simulink model "iwave_dsa_1ant"  (R2019a)
settings: Solver=VariableStepAuto  StartTime=0.0  StopTime=10.0  RelTol=1e-3
undefined symbols (not defined in the file): i
libraries: xbsIndex_r4 x9262, casper_library_misc x249, xps_library x3, casper_library_reorder x2, casper_library_delays x2
(part 15 of 96)

== system iwave_dsa_1ant/pipeline0/input/bus_mux ==
  sel : Inport
  d0 : Inport  Port=2
  d1 : Inport  Port=3
  d2 : Inport  Port=4
  misci : Inport  Port=5
  d_bussify : Subsystem  AncestorBlock=casper_library_flow_control/bus_create  mask(bus_create){inputNum=4}
      mask prompts: inputNum "Number of inputs:"
      mask init:
      | bus_create_init(gcb,...
      |     'inputNum', inputNum);
  dmisc : xbsIndex_r4/Delay  rst=off  infoeditControl=Selection of Reset will increase slice count due to use of real FFs and instead of SRLs  en=off  latency=1  reg_retiming=on  dbl_ovrd=off  block_type=delay
  expand0 : Subsystem  AncestorBlock=casper_library_flow_control/bus_expand  mask(bus_expand){mode=divisions of arbitrary size, outputNum=1, outputWidth=[192;192;192;192], outputBinaryPt=[0  0  0  0], outputArithmeticType=[0  0  0  0], show_format=on, outputToWorkspace=off, variablePrefix=, outputToModelAsWell=on}
      mask prompts: outputNum "Number of outputs:"; outputWidth "Output width [msb ... lsb]:"; outputBinaryPt "Output binary point position [msb ... lsb]:"; outputArithmeticType "Output arithmetic type (ufix=0, fix=1, bool=2) [msb ... lsb]:"; show_format "Print format string?"; outputToWorkspace "Output to workspace?"; variablePrefix "Variable name prefix:"; outputToModelAsWell "Output to model as well?"
      mask help:
      | Expands a 'bus' made using a bus_create or Xilinx
      | concat block.
      | The input will be divided into the specified number
      | of outputs with the specified arithmetic types.
      | Divisions are made from most significant bit.
      mask init: same as iwave_dsa_1ant/pipeline0/bus_expand
      settings: AttributesFormatString=4 outputs: uf192.0,uf192.0,uf192.0,uf192.0,
      mask TypeOptions mode: divisions of equal size | divisions of arbitrary size
      mask Callback mode: bus_expand_callback();
      mask Callback outputWidth: bus_expand_callback();
      mask Callback outputToWorkspace: bus_expand_callback();
  expand1 : Subsystem  AncestorBlock=casper_library_flow_control/bus_expand  mask(bus_expand){mode=divisions of arbitrary size, outputNum=1, outputWidth=[192;192;192;192], outputBinaryPt=[0  0  0  0], outputArithmeticType=[0  0  0  0], show_format=on, outputToWorkspace=off, variablePrefix=, outputToModelAsWell=on}
      mask prompts: outputNum "Number of outputs:"; outputWidth "Output width [msb ... lsb]:"; outputBinaryPt "Output binary point position [msb ... lsb]:"; outputArithmeticType "Output arithmetic type (ufix=0, fix=1, bool=2) [msb ... lsb]:"; show_format "Print format string?"; outputToWorkspace "Output to workspace?"; variablePrefix "Variable name prefix:"; outputToModelAsWell "Output to model as well?"
      mask help:
      | Expands a 'bus' made using a bus_create or Xilinx
      | concat block.
      | The input will be divided into the specified number
      | of outputs with the specified arithmetic types.
      | Divisions are made from most significant bit.
      mask init: same as iwave_dsa_1ant/pipeline0/bus_expand
      settings: AttributesFormatString=4 outputs: uf192.0,uf192.0,uf192.0,uf192.0,
      mask TypeOptions mode: divisions of equal size | divisions of arbitrary size
      mask Callback mode: bus_expand_callback();
      mask Callback outputWidth: bus_expand_callback();
      mask Callback outputToWorkspace: bus_expand_callback();
  expand2 : Subsystem  AncestorBlock=casper_library_flow_control/bus_expand  mask(bus_expand){mode=divisions of arbitrary size, outputNum=1, outputWidth=[192;192;192;192], outputBinaryPt=[0  0  0  0], outputArithmeticType=[0  0  0  0], show_format=on, outputToWorkspace=off, variablePrefix=, outputToModelAsWell=on}
      mask prompts: outputNum "Number of outputs:"; outputWidth "Output width [msb ... lsb]:"; outputBinaryPt "Output binary point position [msb ... lsb]:"; outputArithmeticType "Output arithmetic type (ufix=0, fix=1, bool=2) [msb ... lsb]:"; show_format "Print format string?"; outputToWorkspace "Output to workspace?"; variablePrefix "Variable name prefix:"; outputToModelAsWell "Output to model as well?"
      mask help:
      | Expands a 'bus' made using a bus_create or Xilinx
      | concat block.
      | The input will be divided into the specified number
      | of outputs with the specified arithmetic types.
      | Divisions are made from most significant bit.
      mask init: same as iwave_dsa_1ant/pipeline0/bus_expand
      settings: AttributesFormatString=4 outputs: uf192.0,uf192.0,uf192.0,uf192.0,
      mask TypeOptions mode: divisions of equal size | divisions of arbitrary size
      mask Callback mode: bus_expand_callback();
      mask Callback outputWidth: bus_expand_callback();
      mask Callback outputToWorkspace: bus_expand_callback();
  mux{0..3} (4 alike) : xbsIndex_r4/Mux  inputs=3  en=off  latency=1  precision=Full  arith_type=Unsigned  n_bits=16  bin_pt=14  quantization=Truncate  overflow=Wrap  dbl_ovrd=off  block_type=mux
  sel_expand : Subsystem  AncestorBlock=casper_library_flow_control/bus_expand  mask(bus_expand){mode=divisions of equal size, outputNum=4, outputWidth=2, outputBinaryPt=0, outputArithmeticType=0, show_format=on, outputToWorkspace=off, variablePrefix=, outputToModelAsWell=on}
      mask prompts: outputNum "Number of outputs:"; outputWidth "Output width:"; outputBinaryPt "Output binary point position:"; outputArithmeticType "Output arithmetic type (ufix=0, fix=1, bool=2):"; show_format "Print format string?"; outputToWorkspace "Output to workspace?"; variablePrefix "Variable name prefix:"; outputToModelAsWell "Output to model as well?"
      mask help:
      | Expands a 'bus' made using a bus_create or Xilinx
      | concat block.
      | The input will be divided into the specified number
      | of outputs with the specified arithmetic types.
      | Divisions are made from most significant bit.
      mask init: same as iwave_dsa_1ant/pipeline0/bus_expand
      settings: AttributesFormatString=4 outputs: uf2.0,uf2.0,uf2.0,uf2.0,
      mask TypeOptions mode: divisions of equal size | divisions of arbitrary size
      mask Callback mode: bus_expand_callback();
      mask Callback outputWidth: bus_expand_callback();
      mask Callback outputToWorkspace: bus_expand_callback();
  out : Outport
  misco : Outport  Port=2
  wires:
  sel/1 -> sel_expand/1(bus_in)
  d0/1 -> expand0/1(bus_in)
  d1/1 -> expand1/1(bus_in)
  d2/1 -> expand2/1(bus_in)
  sel_expand/1(msb_out4) -> mux0/1
  expand0/1(msb_out4) -> mux0/2
  expand1/1(msb_out4) -> mux0/3
  expand2/1(msb_out4) -> mux0/4
  sel_expand/2(out3) -> mux1/1
  expand0/2(out3) -> mux1/2
  expand1/2(out3) -> mux1/3
  expand2/2(out3) -> mux1/4
  sel_expand/3(out2) -> mux2/1
  expand0/3(out2) -> mux2/2
  expand1/3(out2) -> mux2/3
  expand2/3(out2) -> mux2/4
  sel_expand/4(lsb_out1) -> mux3/1
  expand0/4(lsb_out1) -> mux3/2
  expand1/4(lsb_out1) -> mux3/3
  expand2/4(lsb_out1) -> mux3/4
  misci/1 -> dmisc/1
  mux0/1 -> d_bussify/1(in1)
  mux1/1 -> d_bussify/2(in2)
  mux2/1 -> d_bussify/3(in3)
  mux3/1 -> d_bussify/4(in4)
  d_bussify/1(bus_out) -> out/1
  dmisc/1 -> misco/1

== system iwave_dsa_1ant/pipeline0/input/rms ==
  note: two clocks after
      | adc_rms_rst goes high
      | the outputs are locked
  note: To provide a means for measuring the magnitude of the signals
      | coming in to each ADC channel, we have a "calc_adc_sum_sq"
      | block which uses a single multiplier, two accumulators, and two
      | regsiters to calculate the sum of 64K ADC samples and the sum
      | of squares of 64K ADC samples.  These can be used to calculate
      | the mean (aka DC offset) and standard deviation (aka RMS) of
      | the ADC inputs.
  note: The sum_sumsq values are Fix_64_0.
      | The upper 29 bits are Fix_29_0 sum of samples.
      | The lower 35 bits are UFix_35_0 sum of squares.
  note: sum,sq,sum,sq,...
  in : Inport
  Constant : Constant  Value=0
  Counter : xbsIndex_r4/Counter  cnt_type=Free Running  cnt_to=Inf  operation=Up  start_count=0  cnt_by_val=1  arith_type=Unsigned  n_bits=16  bin_pt=0  load_pin=off  rst=off  en=off  explicit_period=off  period=1  use_behavioral_HDL=off  implementation=Fabric  use_rpm=on  dbl_ovrd=off  block_type=counter
      settings: xl_area=[0, 0, 0, 0, 0, 0, 0]
  Goto Tag Visibility : GotoTagVisibility  GotoTag=adc_rms_rst
  Slice16 : xbsIndex_r4/Slice  nbits=1  boolean_output=on  mode=Upper Bit Location + Width  bit1=0  base1=MSB of Input  bit0=19  base0=LSB of Input  dbl_ovrd=off  block_type=slice
      settings: infoedit="Extracts a given range of bits from each input sample and presents it at the output.  The output type is ordinarily unsigned with binary point at zero, but can be Boolean when the slice is one bit wide.<P><P>Hardware notes: In hardware this block costs nothing."  block_version=10.1.3
  Subsystem : Subsystem
  Subsystem1 : Subsystem
  Subsystem2 : Subsystem
  Subsystem3 : Subsystem
  Terminator : Terminator
  bram_ctrl : Subsystem
  bus_expand : Subsystem  AncestorBlock=casper_library_flow_control/bus_expand  mask(bus_expand){mode=divisions of equal size, outputNum=8*16, outputWidth=3, outputBinaryPt=0, outputArithmeticType=1, show_format=off, outputToWorkspace=off, variablePrefix=out, outputToModelAsWell=on}
      mask prompts: outputNum "Number of outputs:"; outputWidth "Output width:"; outputBinaryPt "Output binary point position:"; outputArithmeticType "Output arithmetic type (ufix=0, fix=1, bool=2):"; show_format "Print format string?"; outputToWorkspace "Output to workspace?"; variablePrefix "Variable name prefix:"; outputToModelAsWell "Output to model as well?"
      mask help:
      | Expands a 'bus' made using a bus_create or Xilinx
      | concat block.
      | The input will be divided into the specified number
      | of outputs with the specified arithmetic types.
      | Divisions are made from most significant bit.
      mask init: same as iwave_dsa_1ant/pipeline0/bus_expand
      settings: AttributesFormatString=128 outputs
      mask TypeOptions mode: divisions of equal size | divisions of arbitrary size
      mask Callback mode: bus_expand_callback();
      mask Callback outputWidth: bus_expand_callback();
      mask Callback outputToWorkspace: bus_expand_callback();
  edge_detect : Subsystem  AncestorBlock=casper_library_misc/edge_detect  mask(edge_detect){edge=Rising, polarity=Active High, x_in=[0 0.08 0.08 0.16 0.16 0.24 0.24 0.32 0.32 0.4], y_in=[-1 -1  1  1  1  1  1  1  1  1], x_out=[0.6 0.68 0.68 0.76 0.76 0.84 0.84 0.92 0.92 1], y_out=[-1 -1  1  1 -1 -1 -1 -1 -1 -1]}
      mask prompts: edge "Edge Type"; polarity "Output Polarity"; x_in "Input X Positions"; y_in "Input Y Positions"; x_out "Output X Positions"; y_out "Output Y Positions"
      mask help: Output is active for one-cycle after each edge of the specified type (i.e. rising, falling or both).
      mask init: same as iwave_dsa_1ant/pipeline0/sync/ed1
      settings: AttributesFormatString=|
      | rising edges
      | active high
      mask Help: Output is active for one-cycle after each edge of the specified type (i.e. rising, falling, or both).  Latency is zero.
      mask TypeOptions edge: Rising | Falling | Both
      mask TypeOptions polarity: Active High | Active Low
      mask Display:
      | plot(x_in_num,0.5+y_in_num*0.2);
      | plot(x_out_num,0.5+y_out_num*0.2);
  enable : Subsystem  Tag=xps:sw_reg  AncestorBlock=xps_library/Memory/software_register  mask(swreg){io_dir=From Processor, io_delay=0, init_val=0, sample_period=1, names=reg, bitwidths=32, bin_pts=0, arith_types=0, sim_port=on, show_format=off, desc_str=|}
      mask desc_str=|
      | Enable statistics recording. If the least-significant bit
      | is ``1``, statistics will be recorded to RAM.
      mask prompts: io_dir "I/O direction"; io_delay "I/O delay"; init_val "Initial Value"; sample_period "Sample period"; names "Bitfield names [msb...lsb]"; bitwidths "Bitfield widths"; bin_pts "Bitfield binary pts"; arith_types "Bitfield types, ufix=0, fix=1, bool=2"; sim_port "Provide sim input/output?"; show_format "Print format string?"; desc_str "Description"
      mask help: A 32-bit software-accessible register. Can be divided into bitfields of varying widths and types using the fields in the block mask.
      mask init:
      | swreg_init(gcb)
      settings: AttributesFormatString=1input
      mask TypeOptions io_dir: To Processor | From Processor
      mask Callback io_dir:
      | mask_enables = get_param(gcb, 'MaskEnables');
      | mask_names = get_param(gcb, 'MaskNames');
      | if strcmp(get_param(gcb, 'io_dir'), 'To Processor'),
      |     mask_enables{ismember(mask_names, 'sample_period')} = 'off';
      | else
      |     mask_enables{ismember(mask_names, 'sample_period')} = 'on';
      | end
      | set_param(gcb, 'MaskEnables', mask_enables);
      mask DialogControl ParameterTabVar0 Prompt: Setup
  levels : Subsystem  Tag=xps:bram  AncestorBlock=xps_library/Memory/shared_bram  mask{sample_rate=1, init_vals=[0:2^10-1], data_bin_pt=0, optimization=Minimum_Area, reg_core_output=on, reg_prim_output=on, data_width=64, addr_width=9, arith_type=Unsigned, desc_str=|, type_desc=uint64}
      mask desc_str=|
      | Multi-channel statistics. For the ``n`` th 64-bit word, the
      | least signficant 32 bits represent the accumulated
      | ADC power, accumulated over 65536 samples and
      | stored as an unsigned 32-bit integer.
      | The most significant 32 bits represent the sum of
      | 65536 ADC samples stored as a signed 32-bit integer.
      mask prompts: sample_rate "Sample rate"; init_vals "Initial values (simulation only)"; data_bin_pt "Data Binary Point"; reg_core_output "Register Core Output"; reg_prim_output "Register Primitive Output"; data_width "Data Width"; addr_width "Address width"; arith_type "Output Data Type"; desc_str "Description"; type_desc "Word Type Description"
      mask init:
      | shared_bram_mask;
      mask TypeOptions optimization: Minimum_Area | Low_Power
      mask TypeOptions data_width: 8 | 16 | 32 | 64 | 128
      mask TypeOptions arith_type: Unsigned | Signed  (2's comp)
      mask DialogControl Container4 Prompt: Configuration
      mask DialogControl Container10 Prompt: Documentation
  lsb : xbsIndex_r4/Slice  nbits=0  boolean_output=on  mode=Lower Bit Location + Width  bit1=0  base1=MSB of Input  bit0=0  base0=LSB of Input  dbl_ovrd=off  block_type=slice
      settings: block_version=10.1.3
  tag scope: adc_rms_rst=scoped
  wires:
  Counter/1 -> Slice16/1
  Slice16/1 -> edge_detect/1(in)
  edge_detect/1(out) -> [adc_rms_rst]
  enable/1(in_reg) -> lsb/1
  bram_ctrl/1(addr) -> levels/1(addr)
  bram_ctrl/2(data) -> levels/2(data_in)
  bram_ctrl/3(we) -> levels/3(we)
  Constant/1 -> enable/1(sim_1)
  levels/1(data_out) -> Terminator/1
  in/1 -> bus_expand/1(bus_in)
  lsb/1 -> bram_ctrl/1(en)
  Subsystem/1(Out1) -> bram_ctrl/2(adc0)
  Subsystem/2(Out2) -> bram_ctrl/3(adc1)
  Subsystem/3(Out3) -> bram_ctrl/4(adc2)
  Subsystem/4(Out4) -> bram_ctrl/5(adc3)
  Subsystem/5(Out5) -> bram_ctrl/6(adc4)
  Subsystem/6(Out6) -> bram_ctrl/7(adc5)
  Subsystem/7(Out7) -> bram_ctrl/8(adc6)
  Subsystem/8(Out8) -> bram_ctrl/9(adc7)
  Subsystem/9(Out9) -> bram_ctrl/10(adc8)
  Subsystem/10(Out10) -> bram_ctrl/11(adc9)
  Subsystem/11(Out11) -> bram_ctrl/12(adc10)
  Subsystem/12(Out12) -> bram_ctrl/13(adc11)
  Subsystem/13(Out13) -> bram_ctrl/14(adc12)
  Subsystem/14(Out14) -> bram_ctrl/15(adc13)
  Subsystem/15(Out15) -> bram_ctrl/16(adc14)
  Subsystem/16(Out16) -> bram_ctrl/17(adc15)
  Subsystem/17(Out17) -> bram_ctrl/18(adc16)
  Subsystem/18(Out18) -> bram_ctrl/19(adc17)
  Subsystem/19(Out19) -> bram_ctrl/20(adc18)
  Subsystem/20(Out20) -> bram_ctrl/21(adc19)
  Subsystem/21(Out21) -> bram_ctrl/22(adc20)
  Subsystem/22(Out22) -> bram_ctrl/23(adc21)
  Subsystem/23(Out23) -> bram_ctrl/24(adc22)
  Subsystem/24(Out24) -> bram_ctrl/25(adc23)
  Subsystem/25(Out25) -> bram_ctrl/26(adc24)
  Subsystem/26(Out26) -> bram_ctrl/27(adc25)
  Subsystem/27(Out27) -> bram_ctrl/28(adc26)
  Subsystem/28(Out28) -> bram_ctrl/29(adc27)
  Subsystem/29(Out29) -> bram_ctrl/30(adc28)
  Subsystem/30(Out30) -> bram_ctrl/31(adc29)
  Subsystem/31(Out31) -> bram_ctrl/32(adc30)
  Subsystem/32(Out32) -> bram_ctrl/33(adc31)
  bus_expand/1(msb_out128) -> Subsystem/1(In1)
  bus_expand/2(out127) -> Subsystem/2(In2)
  bus_expand/3(out126) -> Subsystem/3(In3)
  bus_expand/4(out125) -> Subsystem/4(In4)
  bus_expand/5(out124) -> Subsystem/5(In5)
  bus_expand/6(out123) -> Subsystem/6(In6)
  bus_expand/7(out122) -> Subsystem/7(In7)
  bus_expand/8(out121) -> Subsystem/8(In8)
  bus_expand/9(out120) -> Subsystem/9(In9)
  bus_expand/10(out119) -> Subsystem/10(In10)
  bus_expand/11(out118) -> Subsystem/11(In11)
  bus_expand/12(out117) -> Subsystem/12(In12)
  bus_expand/13(out116) -> Subsystem/13(In13)
  bus_expand/14(out115) -> Subsystem/14(In14)
  bus_expand/15(out114) -> Subsystem/15(In15)
  bus_expand/16(out113) -> Subsystem/16(In16)
  bus_expand/17(out112) -> Subsystem/17(In17)
  bus_expand/18(out111) -> Subsystem/18(In18)
  bus_expand/19(out110) -> Subsystem/19(In19)
  bus_expand/20(out109) -> Subsystem/20(In20)
  bus_expand/21(out108) -> Subsystem/21(In21)
  bus_expand/22(out107) -> Subsystem/22(In22)
  bus_expand/23(out106) -> Subsystem/23(In23)
  bus_expand/24(out105) -> Subsystem/24(In24)
  bus_expand/25(out104) -> Subsystem/25(In25)
  bus_expand/26(out103) -> Subsystem/26(In26)
  bus_expand/27(out102) -> Subsystem/27(In27)
  bus_expand/28(out101) -> Subsystem/28(In28)
  bus_expand/29(out100) -> Subsystem/29(In29)
  bus_expand/30(out99) -> Subsystem/30(In30)
  bus_expand/31(out98) -> Subsystem/31(In31)
  bus_expand/32(out97) -> Subsystem/32(In32)
  bus_expand/33(out96) -> Subsystem1/1(In1)
  bus_expand/34(out95) -> Subsystem1/2(In2)
  bus_expand/35(out94) -> Subsystem1/3(In3)
  bus_expand/36(out93) -> Subsystem1/4(In4)
  bus_expand/37(out92) -> Subsystem1/5(In5)
  bus_expand/38(out91) -> Subsystem1/6(In6)
  bus_expand/39(out90) -> Subsystem1/7(In7)
  bus_expand/40(out89) -> Subsystem1/8(In8)
  bus_expand/41(out88) -> Subsystem1/9(In9)
  bus_expand/42(out87) -> Subsystem1/10(In10)
  bus_expand/43(out86) -> Subsystem1/11(In11)
  bus_expand/44(out85) -> Subsystem1/12(In12)
  bus_expand/45(out84) -> Subsystem1/13(In13)
  bus_expand/46(out83) -> Subsystem1/14(In14)
  bus_expand/47(out82) -> Subsystem1/15(In15)
  bus_expand/48(out81) -> Subsystem1/16(In16)
  bus_expand/49(out80) -> Subsystem1/17(In17)
  bus_expand/50(out79) -> Subsystem1/18(In18)
  bus_expand/51(out78) -> Subsystem1/19(In19)
  bus_expand/52(out77) -> Subsystem1/20(In20)
  bus_expand/53(out76) -> Subsystem1/21(In21)
  bus_expand/54(out75) -> Subsystem1/22(In22)
  bus_expand/55(out74) -> Subsystem1/23(In23)
  bus_expand/56(out73) -> Subsystem1/24(In24)
  bus_expand/57(out72) -> Subsystem1/25(In25)
  bus_expand/58(out71) -> Subsystem1/26(In26)
  bus_expand/59(out70) -> Subsystem1/27(In27)
  bus_expand/60(out69) -> Subsystem1/28(In28)
  bus_expand/61(out68) -> Subsystem1/29(In29)
  bus_expand/62(out67) -> Subsystem1/30(In30)
  bus_expand/63(out66) -> Subsystem1/31(In31)
  bus_expand/64(out65) -> Subsystem1/32(In32)
  Subsystem1/1(Out1) -> bram_ctrl/34(adc32)
  Subsystem1/2(Out2) -> bram_ctrl/35(adc33)
  Subsystem1/3(Out3) -> bram_ctrl/36(adc34)
  Subsystem1/4(Out4) -> bram_ctrl/37(adc35)
  Subsystem1/5(Out5) -> bram_ctrl/38(adc36)
  Subsystem1/6(Out6) -> bram_ctrl/39(adc37)
  Subsystem1/7(Out7) -> bram_ctrl/40(adc38)
  Subsystem1/8(Out8) -> bram_ctrl/41(adc39)
  Subsystem1/9(Out9) -> bram_ctrl/42(adc40)
  Subsystem1/10(Out10) -> bram_ctrl/43(adc41)
  Subsystem1/11(Out11) -> bram_ctrl/44(adc42)
  Subsystem1/12(Out12) -> bram_ctrl/45(adc43)
  Subsystem1/13(Out13) -> bram_ctrl/46(adc44)
  Subsystem1/14(Out14) -> bram_ctrl/47(adc45)
  Subsystem1/15(Out15) -> bram_ctrl/48(adc46)
  Subsystem1/16(Out16) -> bram_ctrl/49(adc47)
  Subsystem1/17(Out17) -> bram_ctrl/50(adc48)
  Subsystem1/18(Out18) -> bram_ctrl/51(adc49)
  Subsystem1/19(Out19) -> bram_ctrl/52(adc50)
  Subsystem1/20(Out20) -> bram_ctrl/53(adc51)
  Subsystem1/21(Out21) -> bram_ctrl/54(adc52)
  Subsystem1/22(Out22) -> bram_ctrl/55(adc53)
  Subsystem1/23(Out23) -> bram_ctrl/56(adc54)
  Subsystem1/24(Out24) -> bram_ctrl/57(adc55)
  Subsystem1/25(Out25) -> bram_ctrl/58(adc56)
  Subsystem1/26(Out26) -> bram_ctrl/59(adc57)
  Subsystem1/27(Out27) -> bram_ctrl/60(adc58)
  Subsystem1/28(Out28) -> bram_ctrl/61(adc59)
  Subsystem1/29(Out29) -> bram_ctrl/62(adc60)
  Subsystem1/30(Out30) -> bram_ctrl/63(adc61)
  Subsystem1/31(Out31) -> bram_ctrl/64(adc62)
  Subsystem1/32(Out32) -> bram_ctrl/65(adc63)
  bus_expand/65(out64) -> Subsystem2/1(In1)
  bus_expand/66(out63) -> Subsystem2/2(In2)
  bus_expand/67(out62) -> Subsystem2/3(In3)
  bus_expand/68(out61) -> Subsystem2/4(In4)
  bus_expand/69(out60) -> Subsystem2/5(In5)
  bus_expand/70(out59) -> Subsystem2/6(In6)
  bus_expand/71(out58) -> Subsystem2/7(In7)
  bus_expand/72(out57) -> Subsystem2/8(In8)
  bus_expand/73(out56) -> Subsystem2/9(In9)
  bus_expand/74(out55) -> Subsystem2/10(In10)
  bus_expand/75(out54) -> Subsystem2/11(In11)
  bus_expand/76(out53) -> Subsystem2/12(In12)
  bus_expand/77(out52) -> Subsystem2/13(In13)
  bus_expand/78(out51) -> Subsystem2/14(In14)
  bus_expand/79(out50) -> Subsystem2/15(In15)
  bus_expand/80(out49) -> Subsystem2/16(In16)
  bus_expand/81(out48) -> Subsystem2/17(In17)
  bus_expand/82(out47) -> Subsystem2/18(In18)
  bus_expand/83(out46) -> Subsystem2/19(In19)
  bus_expand/84(out45) -> Subsystem2/20(In20)
  bus_expand/85(out44) -> Subsystem2/21(In21)
  bus_expand/86(out43) -> Subsystem2/22(In22)
  bus_expand/87(out42) -> Subsystem2/23(In23)
  bus_expand/88(out41) -> Subsystem2/24(In24)
  bus_expand/89(out40) -> Subsystem2/25(In25)
  bus_expand/90(out39) -> Subsystem2/26(In26)
  bus_expand/91(out38) -> Subsystem2/27(In27)
  bus_expand/92(out37) -> Subsystem2/28(In28)
  bus_expand/93(out36) -> Subsystem2/29(In29)
  bus_expand/94(out35) -> Subsystem2/30(In30)
  bus_expand/95(out34) -> Subsystem2/31(In31)
  bus_expand/96(out33) -> Subsystem2/32(In32)
  Subsystem2/1(Out1) -> bram_ctrl/66(adc64)
  Subsystem2/2(Out2) -> bram_ctrl/67(adc65)
  Subsystem2/3(Out3) -> bram_ctrl/68(adc66)
  Subsystem2/4(Out4) -> bram_ctrl/69(adc67)
  Subsystem2/5(Out5) -> bram_ctrl/70(adc68)
  Subsystem2/6(Out6) -> bram_ctrl/71(adc69)
  Subsystem2/7(Out7) -> bram_ctrl/72(adc70)
  Subsystem2/8(Out8) -> bram_ctrl/73(adc71)
  Subsystem2/9(Out9) -> bram_ctrl/74(adc72)
  Subsystem2/10(Out10) -> bram_ctrl/75(adc73)
  Subsystem2/11(Out11) -> bram_ctrl/76(adc74)
  Subsystem2/12(Out12) -> bram_ctrl/77(adc75)
  Subsystem2/13(Out13) -> bram_ctrl/78(adc76)
  Subsystem2/14(Out14) -> bram_ctrl/79(adc77)
  Subsystem2/15(Out15) -> bram_ctrl/80(adc78)
  Subsystem2/16(Out16) -> bram_ctrl/81(adc79)
  Subsystem2/17(Out17) -> bram_ctrl/82(adc80)
  Subsystem2/18(Out18) -> bram_ctrl/83(adc81)
  Subsystem2/19(Out19) -> bram_ctrl/84(adc82)
  Subsystem2/20(Out20) -> bram_ctrl/85(adc83)
  Subsystem2/21(Out21) -> bram_ctrl/86(adc84)
  Subsystem2/22(Out22) -> bram_ctrl/87(adc85)
  Subsystem2/23(Out23) -> bram_ctrl/88(adc86)
  Subsystem2/24(Out24) -> bram_ctrl/89(adc87)
  Subsystem2/25(Out25) -> bram_ctrl/90(adc88)
  Subsystem2/26(Out26) -> bram_ctrl/91(adc89)
  Subsystem2/27(Out27) -> bram_ctrl/92(adc90)
  Subsystem2/28(Out28) -> bram_ctrl/93(adc91)
  Subsystem2/29(Out29) -> bram_ctrl/94(adc92)
  Subsystem2/30(Out30) -> bram_ctrl/95(adc93)
  Subsystem2/31(Out31) -> bram_ctrl/96(adc94)
  Subsystem2/32(Out32) -> bram_ctrl/97(adc95)
  bus_expand/97(out32) -> Subsystem3/1(In1)
  bus_expand/98(out31) -> Subsystem3/2(In2)
  bus_expand/99(out30) -> Subsystem3/3(In3)
  bus_expand/100(out29) -> Subsystem3/4(In4)
  bus_expand/101(out28) -> Subsystem3/5(In5)
  bus_expand/102(out27) -> Subsystem3/6(In6)
  bus_expand/103(out26) -> Subsystem3/7(In7)
  bus_expand/104(out25) -> Subsystem3/8(In8)
  bus_expand/105(out24) -> Subsystem3/9(In9)
  bus_expand/106(out23) -> Subsystem3/10(In10)
  bus_expand/107(out22) -> Subsystem3/11(In11)
  bus_expand/108(out21) -> Subsystem3/12(In12)
  bus_expand/109(out20) -> Subsystem3/13(In13)
  bus_expand/110(out19) -> Subsystem3/14(In14)
  bus_expand/111(out18) -> Subsystem3/15(In15)
  bus_expand/112(out17) -> Subsystem3/16(In16)
  bus_expand/113(out16) -> Subsystem3/17(In17)
  bus_expand/114(out15) -> Subsystem3/18(In18)
  bus_expand/115(out14) -> Subsystem3/19(In19)
  bus_expand/116(out13) -> Subsystem3/20(In20)
  bus_expand/117(out12) -> Subsystem3/21(In21)
  bus_expand/118(out11) -> Subsystem3/22(In22)
  bus_expand/119(out10) -> Subsystem3/23(In23)
  bus_expand/120(out9) -> Subsystem3/24(In24)
  bus_expand/121(out8) -> Subsystem3/25(In25)
  bus_expand/122(out7) -> Subsystem3/26(In26)
  bus_expand/123(out6) -> Subsystem3/27(In27)
  bus_expand/124(out5) -> Subsystem3/28(In28)
  bus_expand/125(out4) -> Subsystem3/29(In29)
  bus_expand/126(out3) -> Subsystem3/30(In30)
  bus_expand/127(out2) -> Subsystem3/31(In31)
  bus_expand/128(lsb_out1) -> Subsystem3/32(In32)
  Subsystem3/1(Out1) -> bram_ctrl/98(adc96)
  Subsystem3/2(Out2) -> bram_ctrl/99(adc97)
  Subsystem3/3(Out3) -> bram_ctrl/100(adc98)
  Subsystem3/4(Out4) -> bram_ctrl/101(adc99)
  Subsystem3/5(Out5) -> bram_ctrl/102(adc100)
  Subsystem3/6(Out6) -> bram_ctrl/103(adc101)
  Subsystem3/7(Out7) -> bram_ctrl/104(adc102)
  Subsystem3/8(Out8) -> bram_ctrl/105(adc103)
  Subsystem3/9(Out9) -> bram_ctrl/106(adc104)
  Subsystem3/10(Out10) -> bram_ctrl/107(adc105)
  Subsystem3/11(Out11) -> bram_ctrl/108(adc106)
  Subsystem3/12(Out12) -> bram_ctrl/109(adc107)
  Subsystem3/13(Out13) -> bram_ctrl/110(adc108)
  Subsystem3/14(Out14) -> bram_ctrl/111(adc109)
  Subsystem3/15(Out15) -> bram_ctrl/112(adc110)
  Subsystem3/16(Out16) -> bram_ctrl/113(adc111)
  Subsystem3/17(Out17) -> bram_ctrl/114(adc112)
  Subsystem3/18(Out18) -> bram_ctrl/115(adc113)
  Subsystem3/19(Out19) -> bram_ctrl/116(adc114)
  Subsystem3/20(Out20) -> bram_ctrl/117(adc115)
  Subsystem3/21(Out21) -> bram_ctrl/118(adc116)
  Subsystem3/22(Out22) -> bram_ctrl/119(adc117)
  Subsystem3/23(Out23) -> bram_ctrl/120(adc118)
  Subsystem3/24(Out24) -> bram_ctrl/121(adc119)
  Subsystem3/25(Out25) -> bram_ctrl/122(adc120)
  Subsystem3/26(Out26) -> bram_ctrl/123(adc121)
  Subsystem3/27(Out27) -> bram_ctrl/124(adc122)
  Subsystem3/28(Out28) -> bram_ctrl/125(adc123)
  Subsystem3/29(Out29) -> bram_ctrl/126(adc124)
  Subsystem3/30(Out30) -> bram_ctrl/127(adc125)
  Subsystem3/31(Out31) -> bram_ctrl/128(adc126)
  Subsystem3/32(Out32) -> bram_ctrl/129(adc127)

== system iwave_dsa_1ant/pipeline0/input/source_sel0 ==
  sim_1 : Inport
  convert1_1 : DataTypeConversion  OutDataTypeStr=fixdt('ufix32_En0')  LockScale=on
  convert2_1 : DataTypeConversion  OutDataTypeStr=fixdt('ufix32_En0')  ConvertRealWorld=Stored Integer (SI)  LockScale=on
  gain_1 : Gain
  io_delay : xbsIndex_r4/Delay  rst=off  infoeditControl=Selection of Reset will increase slice count due to use of real FFs and instead of SRLs  en=off  latency=0  reg_retiming=on  dbl_ovrd=off  block_type=delay
  iwave_dsa_1ant_test3_pipeline0_input_source_sel0_user_data_out : xbsIndex_r4/Gateway In  gui_display_data_type=Fixed-point  arith_type=Unsigned  n_bits=32  bin_pt=0  preci_type=Single  exp_width=8  frac_width=24  rows=1  columns=1  quantization="Round  (unbiased: +/- Inf)"  overflow=Saturate  period=1  UseAsADC=off  ADCChannel='1'  interface=None  automatic_assignment=on  address_offset=hex2dec('00')  intf_name=''  intf_description=''  default_value=0  timing_constraint=None  locs_specified=off  LOCs={}  io_standard={}  inherit_from_input=off  hdl_port=on  dbl_ovrd=off  block_type=gatewayin
  reint1 : xbsIndex_r4/Reinterpret  force_arith_type=on  arith_type=Unsigned  force_bin_pt=on  bin_pt=0  block_type=reinterpret
  slice_reg : xbsIndex_r4/Slice  nbits=32  boolean_output=off  mode=Lower Bit Location + Width  bit1=0  base1=MSB of Input  bit0=0  base0=LSB of Input  dbl_ovrd=off  block_type=slice
  in_reg : Outport
  wires:
  iwave_dsa_1ant_test3_pipeline0_input_source_sel0_user_data_out/1 -> io_delay/1
  sim_1/1 -> convert1_1/1
  convert1_1/1 -> convert2_1/1
  convert2_1/1 -> gain_1/1
  gain_1/1 -> iwave_dsa_1ant_test3_pipeline0_input_source_sel0_user_data_out/1
  io_delay/1 -> slice_reg/1
  slice_reg/1 -> reint1/1
  reint1/1 -> in_reg/1

== system iwave_dsa_1ant/pipeline0/offset1/bus_create ==
  in1 : Inport
  in2 : Inport  Port=2
  in3 : Inport  Port=3
  in4 : Inport  Port=4
  concatenate : xbsIndex_r4/Concat  num_inputs=4  dbl_ovrd=off  block_type=concat
  reinterpret{1..4} (4 alike) : xbsIndex_r4/Reinterpret  force_arith_type=on  arith_type=Unsigned  force_bin_pt=on  bin_pt=0  block_type=reinterpret
      reinterpret1 settings: infoedit="Changes signal type without altering the binary representation.   You can changed the signal between signed and unsigned, and relocate the binary point.<br><br>Hardware notes: In hardware this block costs nothing.<br><br>Example:  Suppose the input is 6 bits wide, signed, with 2 fractional bits, and the output is forced to unsigned with 0 fractional bits.  Then an input of -2.0 (1110.00 in binary 2's complement) becomes an output of 56 (111000 in binary)."
      reinterpret2 settings: infoedit="Changes signal type without altering the binary representation.   You can changed the signal between signed and unsigned, and relocate the binary point.<br><br>Hardware notes: In hardware this block costs nothing.<br><br>Example:  Suppose the input is 6 bits wide, signed, with 2 fractional bits, and the output is forced to unsigned with 0 fractional bits.  Then an input of -2.0 (1110.00 in binary 2's complement) becomes an output of 56 (111000 in binary)."
  bus_out : Outport
  wires:
  reinterpret4/1 -> concatenate/4
  in4/1 -> reinterpret4/1
  reinterpret3/1 -> concatenate/3
  in3/1 -> reinterpret3/1
  reinterpret2/1 -> concatenate/2
  in2/1 -> reinterpret2/1
  reinterpret1/1 -> concatenate/1
  in1/1 -> reinterpret1/1
  concatenate/1 -> bus_out/1

== system iwave_dsa_1ant/pipeline0/offset1/bus_expand3 ==
  bus_in : Inport
  reinterpret{1..4} (4 alike) : xbsIndex_r4/Reinterpret  force_arith_type=on  arith_type=Unsigned  force_bin_pt=on  bin_pt=0  block_type=reinterpret
  slice1 : xbsIndex_r4/Slice  nbits=128  boolean_output=off  mode=Upper Bit Location + Width  bit1=-384  base1=MSB of Input  bit0=0  base0=LSB of Input  dbl_ovrd=off  block_type=slice
  slice2 : xbsIndex_r4/Slice  nbits=128  boolean_output=off  mode=Upper Bit Location + Width  bit1=-256  base1=MSB of Input  bit0=0  base0=LSB of Input  dbl_ovrd=off  block_type=slice
  slice3 : xbsIndex_r4/Slice  nbits=128  boolean_output=off  mode=Upper Bit Location + Width  bit1=-128  base1=MSB of Input  bit0=0  base0=LSB of Input  dbl_ovrd=off  block_type=slice
  slice4 : xbsIndex_r4/Slice  nbits=128  boolean_output=off  mode=Upper Bit Location + Width  bit1=0  base1=MSB of Input  bit0=0  base0=LSB of Input  dbl_ovrd=off  block_type=slice
  msb_out4 : Outport
  out3 : Outport  Port=2
  out2 : Outport  Port=3
  lsb_out1 : Outport  Port=4
  wires:
  reinterpret1/1 -> lsb_out1/1
  slice1/1 -> reinterpret1/1
  reinterpret2/1 -> out2/1
  slice2/1 -> reinterpret2/1
  reinterpret3/1 -> out3/1
  slice3/1 -> reinterpret3/1
  reinterpret4/1 -> msb_out4/1
  slice4/1 -> reinterpret4/1
  bus_in/1 -> slice1/1, slice2/1, slice3/1, slice4/1

== system iwave_dsa_1ant/pipeline0/offset2/bus_create ==
  in1 : Inport
  in2 : Inport  Port=2
  in3 : Inport  Port=3
  in4 : Inport  Port=4
  concatenate : xbsIndex_r4/Concat  num_inputs=4  dbl_ovrd=off  block_type=concat
  reinterpret{1..4} (4 alike) : xbsIndex_r4/Reinterpret  force_arith_type=on  arith_type=Unsigned  force_bin_pt=on  bin_pt=0  block_type=reinterpret
      reinterpret1 settings: infoedit="Changes signal type without altering the binary representation.   You can changed the signal between signed and unsigned, and relocate the binary point.<br><br>Hardware notes: In hardware this block costs nothing.<br><br>Example:  Suppose the input is 6 bits wide, signed, with 2 fractional bits, and the output is forced to unsigned with 0 fractional bits.  Then an input of -2.0 (1110.00 in binary 2's complement) becomes an output of 56 (111000 in binary)."
      reinterpret2 settings: infoedit="Changes signal type without altering the binary representation.   You can changed the signal between signed and unsigned, and relocate the binary point.<br><br>Hardware notes: In hardware this block costs nothing.<br><br>Example:  Suppose the input is 6 bits wide, signed, with 2 fractional bits, and the output is forced to unsigned with 0 fractional bits.  Then an input of -2.0 (1110.00 in binary 2's complement) becomes an output of 56 (111000 in binary)."
  bus_out : Outport
  wires:
  concatenate/1 -> bus_out/1
  in1/1 -> reinterpret1/1
  reinterpret1/1 -> concatenate/1
  in2/1 -> reinterpret2/1
  reinterpret2/1 -> concatenate/2
  in3/1 -> reinterpret3/1
  reinterpret3/1 -> concatenate/3
  in4/1 -> reinterpret4/1
  reinterpret4/1 -> concatenate/4

== system iwave_dsa_1ant/pipeline0/offset2/bus_expand3 ==
  bus_in : Inport
  reinterpret{1..4} (4 alike) : xbsIndex_r4/Reinterpret  force_arith_type=on  arith_type=Unsigned  force_bin_pt=on  bin_pt=0  block_type=reinterpret
  slice1 : xbsIndex_r4/Slice  nbits=128  boolean_output=off  mode=Upper Bit Location + Width  bit1=-384  base1=MSB of Input  bit0=0  base0=LSB of Input  dbl_ovrd=off  block_type=slice
  slice2 : xbsIndex_r4/Slice  nbits=128  boolean_output=off  mode=Upper Bit Location + Width  bit1=-256  base1=MSB of Input  bit0=0  base0=LSB of Input  dbl_ovrd=off  block_type=slice
  slice3 : xbsIndex_r4/Slice  nbits=128  boolean_output=off  mode=Upper Bit Location + Width  bit1=-128  base1=MSB of Input  bit0=0  base0=LSB of Input  dbl_ovrd=off  block_type=slice
  slice4 : xbsIndex_r4/Slice  nbits=128  boolean_output=off  mode=Upper Bit Location + Width  bit1=0  base1=MSB of Input  bit0=0  base0=LSB of Input  dbl_ovrd=off  block_type=slice
  msb_out4 : Outport
  out3 : Outport  Port=2
  out2 : Outport  Port=3
  lsb_out1 : Outport  Port=4
  wires:
  bus_in/1 -> slice4/1, slice3/1, slice2/1, slice1/1
  slice4/1 -> reinterpret4/1
  reinterpret4/1 -> msb_out4/1
  slice3/1 -> reinterpret3/1
  reinterpret3/1 -> out3/1
  slice2/1 -> reinterpret2/1
  reinterpret2/1 -> out2/1
  slice1/1 -> reinterpret1/1
  reinterpret1/1 -> lsb_out1/1

== system iwave_dsa_1ant/pipeline0/packetizer0/bus_expand ==
  bus_in : Inport
  reinterpret{1..8} (8 alike) : xbsIndex_r4/Reinterpret  force_arith_type=on  arith_type=Unsigned  force_bin_pt=on  bin_pt=0  block_type=reinterpret
  slice1 : xbsIndex_r4/Slice  nbits=1  boolean_output=off  mode=Upper Bit Location + Width  bit1=-7  base1=MSB of Input  bit0=0  base0=LSB of Input  dbl_ovrd=off  block_type=slice
  slice2 : xbsIndex_r4/Slice  nbits=1  boolean_output=off  mode=Upper Bit Location + Width  bit1=-6  base1=MSB of Input  bit0=0  base0=LSB of Input  dbl_ovrd=off  block_type=slice
  slice3 : xbsIndex_r4/Slice  nbits=1  boolean_output=off  mode=Upper Bit Location + Width  bit1=-5  base1=MSB of Input  bit0=0  base0=LSB of Input  dbl_ovrd=off  block_type=slice
  slice4 : xbsIndex_r4/Slice  nbits=1  boolean_output=off  mode=Upper Bit Location + Width  bit1=-4  base1=MSB of Input  bit0=0  base0=LSB of Input  dbl_ovrd=off  block_type=slice
  slice5 : xbsIndex_r4/Slice  nbits=1  boolean_output=off  mode=Upper Bit Location + Width  bit1=-3  base1=MSB of Input  bit0=0  base0=LSB of Input  dbl_ovrd=off  block_type=slice
  slice6 : xbsIndex_r4/Slice  nbits=1  boolean_output=off  mode=Upper Bit Location + Width  bit1=-2  base1=MSB of Input  bit0=0  base0=LSB of Input  dbl_ovrd=off  block_type=slice
  slice7 : xbsIndex_r4/Slice  nbits=1  boolean_output=off  mode=Upper Bit Location + Width  bit1=-1  base1=MSB of Input  bit0=0  base0=LSB of Input  dbl_ovrd=off  block_type=slice
  slice8 : xbsIndex_r4/Slice  nbits=1  boolean_output=off  mode=Upper Bit Location + Width  bit1=0  base1=MSB of Input  bit0=0  base0=LSB of Input  dbl_ovrd=off  block_type=slice
  msb_out8 : Outport
  out7 : Outport  Port=2
  out6 : Outport  Port=3
  out5 : Outport  Port=4
  out4 : Outport  Port=5
  out3 : Outport  Port=6
  out2 : Outport  Port=7
  lsb_out1 : Outport  Port=8
  wires:
  reinterpret1/1 -> lsb_out1/1
  slice1/1 -> reinterpret1/1
  reinterpret2/1 -> out2/1
  slice2/1 -> reinterpret2/1
  reinterpret3/1 -> out3/1
  slice3/1 -> reinterpret3/1
  reinterpret4/1 -> out4/1
  slice4/1 -> reinterpret4/1
  reinterpret5/1 -> out5/1
  slice5/1 -> reinterpret5/1
  reinterpret6/1 -> out6/1
  slice6/1 -> reinterpret6/1
  reinterpret7/1 -> out7/1
  slice7/1 -> reinterpret7/1
  reinterpret8/1 -> msb_out8/1
  slice8/1 -> reinterpret8/1
  bus_in/1 -> slice1/1, slice2/1, slice3/1, slice4/1, slice5/1, slice6/1, slice7/1, slice8/1

== system iwave_dsa_1ant/pipeline0/packetizer0/header ==
  addr : Inport
  data_in : Inport  Port=2
  we : Inport  Port=3
  Terminator : Terminator
  Terminator1 : Terminator
  Terminator2 : Terminator
  adm_pcie_9h7_dts_dual_2x100g_dsp_3b_pipeline0_packetizer0_header_addr : xbsIndex_r4/Gateway Out  inherit_from_input=off  hdl_port=on  rows=1  columns=1  UseAsDAC=off  DACChannel='1'  interface=None  automatic_assignment=on  address_offset=hex2dec('00')  intf_name=''  intf_description=''  timing_constraint=None  locs_specified=off  LOCs={'A5','B9','A9','C1','A3','G6','E9','A6','A7','A8','B8','B1','B3','D9','B5','B4','B6','C2'}  io_standard={}  block_type=gatewayout
      settings: infoedit="Gateway out block.  Converts Xilinx fixed point inputs into ouputs of type Simulink integer, double, or fixed point.<P><P>Hardware notes:  In hardware these blocks become top level output ports or are discarded, depending on how they are configured."  sginterface={'Nallatech'=>{'xdspkit'=>{'non_memory_mapped_port'=>'uprev_Shared_BRAM_addr'}},'Xilinx'=>{'jtaghwcosim'=>{'non_memory_mapped_port'=>'uprev_Shared_BRAM_addr'},'xdspkit'=>{'non_memory_mapped_port'=>'uprev_Shared_BRAM_addr'}}}  xl_area=[0, 0, 0, 0, 0, 0, 0]
  adm_pcie_9h7_dts_dual_2x100g_dsp_3b_pipeline0_packetizer0_header_data_in : xbsIndex_r4/Gateway Out  inherit_from_input=off  hdl_port=on  rows=1  columns=1  UseAsDAC=off  DACChannel='1'  interface=None  automatic_assignment=on  address_offset=hex2dec('00')  intf_name=''  intf_description=''  timing_constraint=None  locs_specified=off  LOCs={'B21','B22','A22','B23','B19','C19','A20','A21','A23','B24','A24','A25','E18','D18','C18','B18'}  io_standard={}  block_type=gatewayout
      settings: infoedit="Gateway out block.  Converts Xilinx fixed point inputs into ouputs of type Simulink integer, double, or fixed point.<P><P>Hardware notes:  In hardware these blocks become top level output ports or are discarded, depending on how they are configured."  sginterface={'Nallatech'=>{'xdspkit'=>{'non_memory_mapped_port'=>'uprev_Shared_BRAM_data_in'}},'Xilinx'=>{'jtaghwcosim'=>{'non_memory_mapped_port'=>'uprev_Shared_BRAM_data_in'},'xdspkit'=>{'non_memory_mapped_port'=>'uprev_Shared_BRAM_data_in'}}}  xl_area=[0, 0, 0, 0, 0, 0, 0]
  adm_pcie_9h7_dts_dual_2x100g_dsp_3b_pipeline0_packetizer0_header_data_out : xbsIndex_r4/Gateway In  gui_display_data_type=Fixed-point  arith_type=Unsigned  n_bits=64  bin_pt=0  preci_type=Single  exp_width=8  frac_width=24  rows=1  columns=1  quantization=Truncate  overflow=Wrap  period=sample_rate  UseAsADC=off  ADCChannel='1'  interface=None  automatic_assignment=on  address_offset=hex2dec('00')  intf_name=''  intf_description=''  default_value=0  timing_constraint=None  locs_specified=off  LOCs={}  io_standard={}  inherit_from_input=off  hdl_port=on  dbl_ovrd=off  block_type=gatewayin
      settings: xl_area=[0, 0, 0, 0, 0, 0, 0]
  adm_pcie_9h7_dts_dual_2x100g_dsp_3b_pipeline0_packetizer0_header_we : xbsIndex_r4/Gateway Out  inherit_from_input=off  hdl_port=on  rows=1  columns=1  UseAsDAC=off  DACChannel='1'  interface=None  automatic_assignment=on  address_offset=hex2dec('00')  intf_name=''  intf_description=''  timing_constraint=None  locs_specified=off  LOCs={'A14'}  io_standard={}  block_type=gatewayout
      settings: infoedit="Gateway out block.  Converts Xilinx fixed point inputs into ouputs of type Simulink integer, double, or fixed point.<P><P>Hardware notes:  In hardware these blocks become top level output ports or are discarded, depending on how they are configured."  xl_area=[0, 0, 0, 0, 0, 0, 0]
  calc_add : Subsystem  mask{data_width=64, addr_width=6, sample_rate=sample_rate}
      mask prompts: data_width "data width"; addr_width "address width"; sample_rate "sample rate"
  convert_addr : xbsIndex_r4/Convert  gui_display_data_type=Fixed-point  arith_type=Unsigned  n_bits=addr_width  bin_pt=0  float_type=Single  exp_bits=8  fraction_bits=24  quantization=Truncate  overflow=Wrap  en=off  latency=0  pipeline=off  dbl_ovrd=off  block_type=convert
      settings: xl_area=[0, 0, 0, 0, 0, 0, 0]
  convert_din1 : xbsIndex_r4/Convert  gui_display_data_type=Fixed-point  arith_type=Unsigned  n_bits=64  bin_pt=0  float_type=Single  exp_bits=8  fraction_bits=24  quantization=Truncate  overflow=Wrap  en=off  latency=0  pipeline=off  dbl_ovrd=off  block_type=convert
      settings: xl_area=[0, 0, 0, 0, 0, 0, 0]
  convert_we : xbsIndex_r4/Convert  gui_display_data_type=Fixed-point  arith_type=Unsigned  n_bits=1  bin_pt=0  float_type=Single  exp_bits=8  fraction_bits=24  quantization=Truncate  overflow=Wrap  en=off  latency=0  pipeline=off  dbl_ovrd=off  block_type=convert
      settings: xl_area=[0, 0, 0, 0, 0, 0, 0]
  munge_in : Subsystem  AncestorBlock=casper_library_flow_control/munge  mask(munge){divisions=2, div_size=[32 32], order=[1  0], arith_type_out=Unsigned, bin_pt_out=0}
      mask prompts: divisions "Number of divisions"; div_size "Division size (bits)"; order "Division packing order"; arith_type_out "Output arithmetic type"; bin_pt_out "Output binary point"
      mask help: Splits an input bus into the specified number of divisions and then recombines them in the order specified (most significant division = 0,least = number divisions-1)
      mask init:
      | munge_init(gcb, ...
      |     'divisions', divisions, ...
      |     'div_size', div_size, ...
      |     'order', order, ...
      |     'arith_type_out', arith_type_out, ...
      |     'bin_pt_out', bin_pt_out);
      settings: AttributesFormatString=|
      | split:[32 32]
      | join:[1 0]
      | Unsigned [64,0]
      mask TypeOptions arith_type_out: Unsigned | Signed  (2's comp) | Floating-point
  munge_out : Subsystem  AncestorBlock=casper_library_flow_control/munge  mask(munge){divisions=2, div_size=[32 32], order=[1  0], arith_type_out=Unsigned, bin_pt_out=0}
      mask prompts: divisions "Number of divisions"; div_size "Division size (bits)"; order "Division packing order"; arith_type_out "Output arithmetic type"; bin_pt_out "Output binary point"
      mask help: Splits an input bus into the specified number of divisions and then recombines them in the order specified (most significant division = 0,least = number divisions-1)
      mask init:
      | munge_init(gcb, ...
      |     'divisions', divisions, ...
      |     'div_size', div_size, ...
      |     'order', order, ...
      |     'arith_type_out', arith_type_out, ...
      |     'bin_pt_out', bin_pt_out);
      settings: AttributesFormatString=|
      | split:[32 32]
      | join:[1 0]
      | Unsigned [64,0]
      mask TypeOptions arith_type_out: Unsigned | Signed  (2's comp) | Floating-point
  sim_mem : Subsystem  mask{arith_type=Unsigned, addr_width=npol_bits + nchan_bits - nparallel_bits - step_bits, data_width=64, data_bin_pt=0, init_vals=[117440512          0          0          0          0          0          0          0          0          0          0          0          0          0          0          0          0          0          0          0          0          0          0          0          0          0          0          0          0          0          0          0          0          0          0          0          0          0          0          0          0          0          0          0          0          0          0          0          0          0          0          0          0          0          0          0          0          0          0          0          0          0          0          0], sample_rate=1, csp_latency=1}
      mask prompts: arith_type "Output Data Type"; addr_width "Address width"; data_width "Data width"; data_bin_pt "Data Binary Point"; init_vals "Initial values"; sample_rate "Sample rate"; csp_latency "Latency"
      mask init:
      | % set_param([gcb, '/data_to_xilinx'], 'arith_type', arith_type)
      | % set_param([gcb, '/data_to_xilinx'], 'n_bits', get_param(gcb, 'data_width'))
      mask TypeOptions arith_type: Unsigned | Signed  (2's comp)
      mask TypeOptions data_width: 8 | 16 | 32 | 64 | 128
  data_out : Outport
  wires:
  munge_in/1(dout) -> convert_din1/1, sim_mem/2(data)
  we/1 -> convert_we/1, sim_mem/3(we)
  addr/1 -> calc_add/1(in)
  convert_we/1 -> adm_pcie_9h7_dts_dual_2x100g_dsp_3b_pipeline0_packetizer0_header_we/1
  adm_pcie_9h7_dts_dual_2x100g_dsp_3b_pipeline0_packetizer0_header_addr/1 -> Terminator/1
  adm_pcie_9h7_dts_dual_2x100g_dsp_3b_pipeline0_packetizer0_header_data_in/1 -> Terminator1/1
  adm_pcie_9h7_dts_dual_2x100g_dsp_3b_pipeline0_packetizer0_header_we/1 -> Terminator2/1
  calc_add/1(out) -> convert_addr/1, sim_mem/1(addr)
  data_in/1 -> munge_in/1(din)
  convert_din1/1 -> adm_pcie_9h7_dts_dual_2x100g_dsp_3b_pipeline0_packetizer0_header_data_in/1
  convert_addr/1 -> adm_pcie_9h7_dts_dual_2x100g_dsp_3b_pipeline0_packetizer0_header_addr/1
  adm_pcie_9h7_dts_dual_2x100g_dsp_3b_pipeline0_packetizer0_header_data_out/1 -> munge_out/1(din)
  sim_mem/1(data_out) -> adm_pcie_9h7_dts_dual_2x100g_dsp_3b_pipeline0_packetizer0_header_data_out/1
  munge_out/1(dout) -> data_out/1
